simulink library "halout"  (R2021b)
settings: Solver=VariableStepAuto  StartTime=0.0  StopTime=10.0  RelTol=1e-3
undefined symbols (not defined in the file): C_TASK_5MS_S, KHAL_CAN1TxReq_flg, KHAL_CAN2TxReq_flg, KHAL_CAN3TxReq_flg, KHAL_CAN4TxReq_flg, KHAL_CAN5TxReq_flg, KHAL_CAN6TxReq_flg, KHAL_CAN7TxReq_flg, TRUE
libraries: FVT_lib x65, simulink x6
(part 6 of 6)

== system halout/HAL_OUT/CAN4/FD4_CE100_0_0x209/FDCBCMMDCloseSVCmd ==
  FDCBCMMDCloseSVCmd : Inport
  Data Type Conversion : DataTypeConversion  OutDataTypeStr=uint8  RndMeth=Round
  CAN4_FDC_BCM_MDCloseSV_Cmd : Outport
  wires:
  Data Type Conversion/1 -> CAN4_FDC_BCM_MDCloseSV_Cmd/1
  FDCBCMMDCloseSVCmd/1 -> Data Type Conversion/1

== system halout/HAL_OUT/CAN4/FD4_CE100_0_0x209/FDCBCMMDOpenSVCmd ==
  FDCBCMMDOpenSVCmd : Inport
  Data Type Conversion : DataTypeConversion  OutDataTypeStr=uint8  RndMeth=Round
  CAN4_FDC_BCM_MDOpenSV_Cmd : Outport
  wires:
  Data Type Conversion/1 -> CAN4_FDC_BCM_MDOpenSV_Cmd/1
  FDCBCMMDOpenSVCmd/1 -> Data Type Conversion/1

== system halout/HAL_OUT/CAN4/FD4_CE100_0_0x209/FDCBCMMDoorSta ==
  FDCBCMMDoorSta : Inport
  Data Type Conversion : DataTypeConversion  OutDataTypeStr=uint8  RndMeth=Round
  CAN4_FDC_BCM_MDoor_Sta : Outport
  wires:
  Data Type Conversion/1 -> CAN4_FDC_BCM_MDoor_Sta/1
  FDCBCMMDoorSta/1 -> Data Type Conversion/1

== system halout/HAL_OUT/CAN4/FD4_CE100_0_0x209/FDCBCMOutDoorOpenSWSta ==
  FDCBCMOutDoorOpenSWSta : Inport
  Data Type Conversion : DataTypeConversion  OutDataTypeStr=uint8  RndMeth=Round
  CAN4_FDC_BCM_OutDoorOpenSW_Sta : Outport
  wires:
  Data Type Conversion/1 -> CAN4_FDC_BCM_OutDoorOpenSW_Sta/1
  FDCBCMOutDoorOpenSWSta/1 -> Data Type Conversion/1

== system halout/HAL_OUT/CAN4/FD4_CE100_0_0x209/FDCBCMPLampCmd ==
  FDCBCMPLampCmd : Inport
  Data Type Conversion : DataTypeConversion  OutDataTypeStr=uint8  RndMeth=Round
  CAN4_FDC_BCM_PLamp_Cmd : Outport
  wires:
  Data Type Conversion/1 -> CAN4_FDC_BCM_PLamp_Cmd/1
  FDCBCMPLampCmd/1 -> Data Type Conversion/1

== system halout/HAL_OUT/CAN4/FD4_CE100_0_0x209/FDCBCMRBSDRCmd ==
  FDCBCMRBSDRCmd : Inport
  Data Type Conversion : DataTypeConversion  OutDataTypeStr=uint8  RndMeth=Round
  CAN4_FDC_BCM_RBSDR_Cmd : Outport
  wires:
  Data Type Conversion/1 -> CAN4_FDC_BCM_RBSDR_Cmd/1
  FDCBCMRBSDRCmd/1 -> Data Type Conversion/1

== system halout/HAL_OUT/CAN4/FD4_CE100_0_0x209/FDCBCMRBSDYCmd ==
  FDCBCMRBSDYCmd : Inport
  Data Type Conversion : DataTypeConversion  OutDataTypeStr=uint8  RndMeth=Round
  CAN4_FDC_BCM_RBSDY_Cmd : Outport
  wires:
  Data Type Conversion/1 -> CAN4_FDC_BCM_RBSDY_Cmd/1
  FDCBCMRBSDYCmd/1 -> Data Type Conversion/1

== system halout/HAL_OUT/CAN4/FD4_CE100_0_0x209/FDCBCMRDRLCmd ==
  FDCBCMRDRLCmd : Inport
  Data Type Conversion : DataTypeConversion  OutDataTypeStr=uint8  RndMeth=Round
  CAN4_FDC_BCM_RDRL_Cmd : Outport
  wires:
  Data Type Conversion/1 -> CAN4_FDC_BCM_RDRL_Cmd/1
  FDCBCMRDRLCmd/1 -> Data Type Conversion/1

== system halout/HAL_OUT/CAN4/FD4_CE100_0_0x209/FDCBCMRDoorSta ==
  FDCBCMRDoorSta : Inport
  Data Type Conversion : DataTypeConversion  OutDataTypeStr=uint8  RndMeth=Round
  CAN4_FDC_BCM_RDoor_Sta : Outport
  wires:
  Data Type Conversion/1 -> CAN4_FDC_BCM_RDoor_Sta/1
  FDCBCMRDoorSta/1 -> Data Type Conversion/1

== system halout/HAL_OUT/CAN4/FD4_CE100_0_0x209/FDCBCMRFLampCmd ==
  FDCBCMRFLampCmd : Inport
  Data Type Conversion : DataTypeConversion  OutDataTypeStr=uint8  RndMeth=Round
  CAN4_FDC_BCM_RFLamp_Cmd : Outport
  wires:
  Data Type Conversion/1 -> CAN4_FDC_BCM_RFLamp_Cmd/1
  FDCBCMRFLampCmd/1 -> Data Type Conversion/1

== system halout/HAL_OUT/CAN4/FD4_CE100_0_0x209/FDCBCMRGearSta ==
  FDCBCMRGearSta : Inport
  Data Type Conversion : DataTypeConversion  OutDataTypeStr=uint8  RndMeth=Round
  CAN4_FDC_BCM_RGear_Sta : Outport
  wires:
  Data Type Conversion/1 -> CAN4_FDC_BCM_RGear_Sta/1
  FDCBCMRGearSta/1 -> Data Type Conversion/1

== system halout/HAL_OUT/CAN4/FD4_CE100_0_0x209/FDCBCMRTurnLpCmd ==
  FDCBCMRTurnLpCmd : Inport
  Data Type Conversion : DataTypeConversion  OutDataTypeStr=uint8  RndMeth=Round
  CAN4_FDC_BCM_RTurnLp_Cmd : Outport
  wires:
  Data Type Conversion/1 -> CAN4_FDC_BCM_RTurnLp_Cmd/1
  FDCBCMRTurnLpCmd/1 -> Data Type Conversion/1

== system halout/HAL_OUT/CAN4/FD4_CE100_0_0x209/FDCBCMRoomLpAmbCmd ==
  FDCBCMRoomLpAmbCmd : Inport
  Data Type Conversion : DataTypeConversion  OutDataTypeStr=uint8  RndMeth=Round
  CAN4_FDC_BCM_RoomLpAmb_Cmd : Outport
  wires:
  Data Type Conversion/1 -> CAN4_FDC_BCM_RoomLpAmb_Cmd/1
  FDCBCMRoomLpAmbCmd/1 -> Data Type Conversion/1

== system halout/HAL_OUT/CAN4/FD4_CE100_0_0x209/FDCBCMSLTLpCmd ==
  FDCBCMSLTLpCmd : Inport
  Data Type Conversion : DataTypeConversion  OutDataTypeStr=uint8  RndMeth=Round
  CAN4_FDC_BCM_SLTLp_Cmd : Outport
  wires:
  Data Type Conversion/1 -> CAN4_FDC_BCM_SLTLp_Cmd/1
  FDCBCMSLTLpCmd/1 -> Data Type Conversion/1

== system halout/HAL_OUT/CAN4/FD4_CE100_0_0x209/FDCBCMSMKLCmd ==
  FDCBCMSMKLCmd : Inport
  Data Type Conversion : DataTypeConversion  OutDataTypeStr=uint8  RndMeth=Round
  CAN4_FDC_BCM_SMKL_Cmd : Outport
  wires:
  Data Type Conversion/1 -> CAN4_FDC_BCM_SMKL_Cmd/1
  FDCBCMSMKLCmd/1 -> Data Type Conversion/1

== system halout/HAL_OUT/CAN4/FD4_CE100_0_0x209/FDCBCMSMKRCmd ==
  FDCBCMSMKRCmd : Inport
  Data Type Conversion : DataTypeConversion  OutDataTypeStr=uint8  RndMeth=Round
  CAN4_FDC_BCM_SMKR_Cmd : Outport
  wires:
  Data Type Conversion/1 -> CAN4_FDC_BCM_SMKR_Cmd/1
  FDCBCMSMKRCmd/1 -> Data Type Conversion/1

== system halout/HAL_OUT/CAN4/FD4_CE100_0_0x209/FDCBCMSRTLpCmd ==
  FDCBCMSRTLpCmd : Inport
  Data Type Conversion : DataTypeConversion  OutDataTypeStr=uint8  RndMeth=Round
  CAN4_FDC_BCM_SRTLp_Cmd : Outport
  wires:
  Data Type Conversion/1 -> CAN4_FDC_BCM_SRTLp_Cmd/1
  FDCBCMSRTLpCmd/1 -> Data Type Conversion/1

== system halout/HAL_OUT/CAN4/FD4_CE100_0_0x209/FDCBCMSTOPBALLCmd ==
  FDCBCMSTOPBALLCmd : Inport
  Data Type Conversion : DataTypeConversion  OutDataTypeStr=uint8  RndMeth=Round
  CAN4_FDC_BCM_STOPBALL_Cmd : Outport
  wires:
  Data Type Conversion/1 -> CAN4_FDC_BCM_STOPBALL_Cmd/1
  FDCBCMSTOPBALLCmd/1 -> Data Type Conversion/1

== system halout/HAL_OUT/CAN4/FD4_CE100_0_0x209/FDCBCMStopINDCmd ==
  FDCBCMStopINDCmd : Inport
  Data Type Conversion : DataTypeConversion  OutDataTypeStr=uint8  RndMeth=Round
  CAN4_FDC_BCM_Stop_IND_Cmd : Outport
  wires:
  Data Type Conversion/1 -> CAN4_FDC_BCM_Stop_IND_Cmd/1
  FDCBCMStopINDCmd/1 -> Data Type Conversion/1

== system halout/HAL_OUT/CAN4/FD4_CE100_0_0x209/FDCBCMTurnLpPatternSta ==
  FDCBCMTurnLpPatternSta : Inport
  Data Type Conversion : DataTypeConversion  OutDataTypeStr=uint8  RndMeth=Round
  CAN4_FDC_BCM_TurnLpPattern_Sta : Outport
  wires:
  Data Type Conversion/1 -> CAN4_FDC_BCM_TurnLpPattern_Sta/1
  FDCBCMTurnLpPatternSta/1 -> Data Type Conversion/1

== system halout/HAL_OUT/CAN4/FD4_CE100_0_0x209/FDCBCMWasherCmd ==
  FDCBCMWasherCmd : Inport
  Data Type Conversion : DataTypeConversion  OutDataTypeStr=uint8  RndMeth=Round
  CAN4_FDC_BCM_Washer_Cmd : Outport
  wires:
  Data Type Conversion/1 -> CAN4_FDC_BCM_Washer_Cmd/1
  FDCBCMWasherCmd/1 -> Data Type Conversion/1

== system halout/HAL_OUT/CAN4/FD4_CE100_0_0x209/FDCBCMWiperHCmd ==
  FDCBCMWiperHCmd : Inport
  Data Type Conversion : DataTypeConversion  OutDataTypeStr=uint8  RndMeth=Round
  CAN4_FDC_BCM_WiperH_Cmd : Outport
  wires:
  Data Type Conversion/1 -> CAN4_FDC_BCM_WiperH_Cmd/1
  FDCBCMWiperHCmd/1 -> Data Type Conversion/1

== system halout/HAL_OUT/CAN4/FD4_CE100_0_0x209/FDCBCMWiperLCmd ==
  FDCBCMWiperLCmd : Inport
  Data Type Conversion : DataTypeConversion  OutDataTypeStr=uint8  RndMeth=Round
  CAN4_FDC_BCM_WiperL_Cmd : Outport
  wires:
  Data Type Conversion/1 -> CAN4_FDC_BCM_WiperL_Cmd/1
  FDCBCMWiperLCmd/1 -> Data Type Conversion/1

== system halout/HAL_OUT/CAN4/FD4_CE100_0_0x209/VCUKeyStatus ==
  VCUKeyStatus : Inport
  Data Type Conversion : DataTypeConversion  OutDataTypeStr=uint8  RndMeth=Round
  CAN4_VCUKeyStatus : Outport
  wires:
  Data Type Conversion/1 -> CAN4_VCUKeyStatus/1
  VCUKeyStatus/1 -> Data Type Conversion/1

== system halout/HAL_OUT/CAN4/FD4_CE100_1_0x210/FDCBCMFRoomLpCmd ==
  FDCBCMFRoomLpCmd : Inport
  Data Type Conversion : DataTypeConversion  OutDataTypeStr=uint8  RndMeth=Round
  CAN4_FDC_BCM_FRoomLp_Cmd : Outport
  wires:
  Data Type Conversion/1 -> CAN4_FDC_BCM_FRoomLp_Cmd/1
  FDCBCMFRoomLpCmd/1 -> Data Type Conversion/1

== system halout/HAL_OUT/CAN4/FD4_CE100_1_0x210/FDCBCMMRoomLpCmd ==
  FDCBCMMRoomLpCmd : Inport
  Data Type Conversion : DataTypeConversion  OutDataTypeStr=uint8  RndMeth=Round
  CAN4_FDC_BCM_MRoomLp_Cmd : Outport
  wires:
  Data Type Conversion/1 -> CAN4_FDC_BCM_MRoomLp_Cmd/1
  FDCBCMMRoomLpCmd/1 -> Data Type Conversion/1

== system halout/HAL_OUT/CAN4/FD4_CE100_1_0x210/FDCBCMRRoomLpCmd ==
  FDCBCMRRoomLpCmd : Inport
  Data Type Conversion : DataTypeConversion  OutDataTypeStr=uint8  RndMeth=Round
  CAN4_FDC_BCM_RRoomLp_Cmd : Outport
  wires:
  Data Type Conversion/1 -> CAN4_FDC_BCM_RRoomLp_Cmd/1
  FDCBCMRRoomLpCmd/1 -> Data Type Conversion/1

== system halout/HAL_OUT/CAN4/FD4_CE100_1_0x210/FDCTHCMCoolFanReqCmd ==
  FDCTHCMCoolFanReqCmd : Inport
  Data Type Conversion : DataTypeConversion  OutDataTypeStr=uint8  RndMeth=Round
  convert_out : FVT_lib/hal/convert_out  gain=0.5  offset=0
  CAN4_FDC_THCM_CoolFanReq_Cmd : Outport
  wires:
  Data Type Conversion/1 -> CAN4_FDC_THCM_CoolFanReq_Cmd/1
  convert_out/1 -> Data Type Conversion/1
  FDCTHCMCoolFanReqCmd/1 -> convert_out/1

== system halout/HAL_OUT/CAN5/FD5_C100_0_0x18F348D0/AlcLockSta ==
  AlcLockSta : Inport
  Data Type Conversion : DataTypeConversion  OutDataTypeStr=uint8  RndMeth=Round
  CAN5_AlcLockSta : Outport
  wires:
  Data Type Conversion/1 -> CAN5_AlcLockSta/1
  AlcLockSta/1 -> Data Type Conversion/1

== system halout/HAL_OUT/CAN5/FD5_C100_0_0x18F348D0/B2VAPlusSta ==
  B2VAPlusSta : Inport
  Data Type Conversion : DataTypeConversion  OutDataTypeStr=uint8  RndMeth=Round
  CAN5_B2VAPlusSta : Outport
  wires:
  Data Type Conversion/1 -> CAN5_B2VAPlusSta/1
  B2VAPlusSta/1 -> Data Type Conversion/1

== system halout/HAL_OUT/CAN5/FD5_C100_0_0x18F348D0/VCUHVILSta ==
  VCUHVILSta : Inport
  Data Type Conversion : DataTypeConversion  OutDataTypeStr=uint8  RndMeth=Round
  CAN5_VCUHVILSta : Outport
  wires:
  Data Type Conversion/1 -> CAN5_VCUHVILSta/1
  VCUHVILSta/1 -> Data Type Conversion/1

== system halout/HAL_OUT/CAN5/FD5_C200_0_0x20D/SysPowerMode ==
  SysPowerMode : Inport
  Data Type Conversion : DataTypeConversion  OutDataTypeStr=uint8  RndMeth=Round
  CAN5_SysPowerMode : Outport
  wires:
  Data Type Conversion/1 -> CAN5_SysPowerMode/1
  SysPowerMode/1 -> Data Type Conversion/1

== system halout/HAL_OUT/CAN6/FD6_C200_0_0x20C/SysPowerMode ==
  SysPowerMode : Inport
  Data Type Conversion : DataTypeConversion  OutDataTypeStr=uint8  RndMeth=Round
  CAN6_SysPowerMode : Outport
  wires:
  Data Type Conversion/1 -> CAN6_SysPowerMode/1
  SysPowerMode/1 -> Data Type Conversion/1

== system halout/HAL_OUT/CAN7/FD7_C100_0_0x19F005D0/VCUKeyStatus ==
  VCUKeyStatus : Inport
  Data Type Conversion : DataTypeConversion  OutDataTypeStr=uint8  RndMeth=Round
  CAN7_VCUKeyStatus : Outport
  wires:
  Data Type Conversion/1 -> CAN7_VCUKeyStatus/1
  VCUKeyStatus/1 -> Data Type Conversion/1

== system halout/HAL_OUT/CAN7/FD7_C10_0_0xC61D0D1/EMotorSpd ==
  EMotorSpd : Inport
  Data Type Conversion : DataTypeConversion  OutDataTypeStr=uint16  RndMeth=Round
  CAN7_EMotorSpd : Outport
  wires:
  Data Type Conversion/1 -> CAN7_EMotorSpd/1
  EMotorSpd/1 -> Data Type Conversion/1

== system halout/HAL_OUT/CAN7/FD7_C200_0_0x18F003EF/SysPowerMode ==
  SysPowerMode : Inport
  Data Type Conversion : DataTypeConversion  OutDataTypeStr=uint8  RndMeth=Round
  CAN7_SysPowerMode : Outport
  wires:
  Data Type Conversion/1 -> CAN7_SysPowerMode/1
  SysPowerMode/1 -> Data Type Conversion/1

== system halout/HAL_OUT/CAN7/FD7_C50_0_0xCF00300/AccPedalPos1 ==
  AccPedalPos1 : Inport
  Data Type Conversion : DataTypeConversion  OutDataTypeStr=uint8  RndMeth=Round
  convert_out : FVT_lib/hal/convert_out  gain=0.4  offset=0
  CAN7_AccPedalPos1 : Outport
  wires:
  Data Type Conversion/1 -> CAN7_AccPedalPos1/1
  convert_out/1 -> Data Type Conversion/1
  AccPedalPos1/1 -> convert_out/1

== system halout/HAL_OUT/CAN7/FD7_CE100_0_0x18FA05B9/FDCBCMDVRSignalLCmd ==
  FDCBCMDVRSignalLCmd : Inport
  Data Type Conversion : DataTypeConversion  OutDataTypeStr=uint8  RndMeth=Round
  CAN7_FDC_BCM_DVRSignalL_Cmd : Outport
  wires:
  Data Type Conversion/1 -> CAN7_FDC_BCM_DVRSignalL_Cmd/1
  FDCBCMDVRSignalLCmd/1 -> Data Type Conversion/1

== system halout/HAL_OUT/CAN7/FD7_CE100_0_0x18FA05B9/FDCBCMDVRSignalRCmd ==
  FDCBCMDVRSignalRCmd : Inport
  Data Type Conversion : DataTypeConversion  OutDataTypeStr=uint8  RndMeth=Round
  CAN7_FDC_BCM_DVRSignalR_Cmd : Outport
  wires:
  Data Type Conversion/1 -> CAN7_FDC_BCM_DVRSignalR_Cmd/1
  FDCBCMDVRSignalRCmd/1 -> Data Type Conversion/1

== system halout/HAL_OUT/CAN7/FD7_CE100_0_0x18FA05B9/FDCBCMFDoorSta ==
  FDCBCMFDoorSta : Inport
  Data Type Conversion : DataTypeConversion  OutDataTypeStr=uint8  RndMeth=Round
  CAN7_FDC_BCM_FDoor_Sta : Outport
  wires:
  Data Type Conversion/1 -> CAN7_FDC_BCM_FDoor_Sta/1
  FDCBCMFDoorSta/1 -> Data Type Conversion/1

== system halout/HAL_OUT/CAN7/FD7_CE100_0_0x18FA05B9/FDCBCMHBeamCmd ==
  FDCBCMHBeamCmd : Inport
  Data Type Conversion : DataTypeConversion  OutDataTypeStr=uint8  RndMeth=Round
  CAN7_FDC_BCM_HBeam_Cmd : Outport
  wires:
  Data Type Conversion/1 -> CAN7_FDC_BCM_HBeam_Cmd/1
  FDCBCMHBeamCmd/1 -> Data Type Conversion/1

== system halout/HAL_OUT/CAN7/FD7_CE100_0_0x18FA05B9/FDCBCMLBeamCmd ==
  FDCBCMLBeamCmd : Inport
  Data Type Conversion : DataTypeConversion  OutDataTypeStr=uint8  RndMeth=Round
  CAN7_FDC_BCM_LBeam_Cmd : Outport
  wires:
  Data Type Conversion/1 -> CAN7_FDC_BCM_LBeam_Cmd/1
  FDCBCMLBeamCmd/1 -> Data Type Conversion/1

== system halout/HAL_OUT/CAN7/FD7_CE100_0_0x18FA05B9/FDCBCMMDoorSta ==
  FDCBCMMDoorSta : Inport
  Data Type Conversion : DataTypeConversion  OutDataTypeStr=uint8  RndMeth=Round
  CAN7_FDC_BCM_MDoor_Sta : Outport
  wires:
  Data Type Conversion/1 -> CAN7_FDC_BCM_MDoor_Sta/1
  FDCBCMMDoorSta/1 -> Data Type Conversion/1

== system halout/HAL_OUT/CAN7/FD7_CE100_0_0x18FA05B9/FDCBCMPLampCmd ==
  FDCBCMPLampCmd : Inport
  Data Type Conversion : DataTypeConversion  OutDataTypeStr=uint8  RndMeth=Round
  CAN7_FDC_BCM_PLamp_Cmd : Outport
  wires:
  Data Type Conversion/1 -> CAN7_FDC_BCM_PLamp_Cmd/1
  FDCBCMPLampCmd/1 -> Data Type Conversion/1

== stateflow chart halout/HAL_OUT/CAN3/FD3_VCU2_Tx/Chart ==
  state TrigCounter
    en:
    counter = 0;
    counter++;
    (default) -> (junction 5)
    TrigCounter -> (junction 5) : {
        | counter++;
        | }
    (junction 5) -> (junction 6) [order 1] : [TxReq && (counter %% CycleCnt) == 0]
    (junction 5) -> (junction 7) [order 2]
    (junction 6) -> (junction 8) : {
        | TxTrigger;
        | counter = 0;
        | }
    (junction 8) -> (junction 7)
    (junction 7) -> (junction 34)
    (junction 34) -> (junction 33) [order 1] : [ !TxReq]
    (junction 34) -> (junction 35) [order 2]
    (junction 33) -> (junction 36) : {
        | counter = 0;
        | }
    (junction 36) -> (junction 35)
    (junction 35) -> (junction 44)
  data: TxReq input; CycleCnt input; counter local uint16
  events: TxTrigger output FUNCTION_CALL_EVENT

== stateflow chart halout/HAL_OUT/CAN3/FD3_C10_1_0xCFF05EF/CRC_TX/Checksum_J1939_SPN4207 ==
  (default) -> (junction 2) : {
      | ChecksumLocal = (Byte1+Byte2+Byte3+Byte4+Byte5+Byte6+Byte7)...
      | +(MsgCntLocal & 0x0F)...
      | + (MsgIDLowByte + MsgIDMidLowByte + MsgIDMidHighByte + MsgIDHighByte);
      | }
  (junction 2) -> (junction 5)
  (junction 5) -> (junction 7) : {
      | MsgChecksumLocal = (((ChecksumLocal>>6) & 0x03)...
      | + (ChecksumLocal>>3)...
      | + ChecksumLocal)...
      | & 0x07;
      | }
  data: Byte1 input; Byte2 input; Byte3 input; Byte4 input; Byte5 input; Byte6 input; Byte7 input; MsgCntLocal input; MsgIDLowByte input; MsgIDMidLowByte input; MsgIDMidHighByte input; MsgIDHighByte input; MsgChecksumLocal output uint8; ChecksumLocal local single

== stateflow chart halout/HAL_OUT/CAN3/FD3_C10_1_0xCFF05EF/CRC_TX/Rolling_Counter ==
  state RollingCounter
    en:
    MsgCntLocal = 0;
    RollingCounter -> (junction 2) : {MsgCntLocal ++;}
    (junction 2) -> (junction 4) [order 1] : [MsgCntLocal > 0x07]
    (junction 2) -> (junction 6) [order 2]
    (junction 4) -> (junction 8) : {MsgCntLocal = 0;}
  data: MsgCntLocal output uint8

== stateflow chart halout/HAL_OUT/CAN_Scheduler ==
  state CAN_scheduler
    (default) -> (junction 55)
    CAN_scheduler -> (junction 55)
    (junction 55) -> (junction 53) [order 1] : [KHAL_CAN1TxReq_flg && VOUTP_ALLCANTxReq_flg]
    (junction 55) -> (junction 214) [order 2]
    (junction 53) -> (junction 212) : {
        | trig_can1;
        | }
    (junction 212) -> (junction 214)
    (junction 214) -> (junction 250)
    (junction 250) -> (junction 251) [order 1] : [KHAL_CAN2TxReq_flg && VOUTP_ALLCANTxReq_flg]
    (junction 250) -> (junction 253) [order 2]
    (junction 251) -> (junction 247) : {
        | trig_can2;
        | }
    (junction 247) -> (junction 253)
    (junction 253) -> (junction 258)
    (junction 258) -> (junction 259) [order 1] : [KHAL_CAN3TxReq_flg && VOUTP_ALLCANTxReq_flg]
    (junction 258) -> (junction 261) [order 2]
    (junction 259) -> (junction 255) : {
        | trig_can3;
        | }
    (junction 255) -> (junction 261)
    (junction 261) -> (junction 266)
    (junction 266) -> (junction 267) [order 1] : [KHAL_CAN4TxReq_flg && VOUTP_ALLCANTxReq_flg]
    (junction 266) -> (junction 269) [order 2]
    (junction 267) -> (junction 263) : {
        | trig_can4;
        | }
    (junction 263) -> (junction 269)
    (junction 269) -> (junction 274)
    (junction 274) -> (junction 275) [order 1] : [KHAL_CAN5TxReq_flg && VOUTP_ALLCANTxReq_flg]
    (junction 274) -> (junction 277) [order 2]
    (junction 275) -> (junction 271) : {
        | trig_can5;
        | }
    (junction 271) -> (junction 277)
    (junction 277) -> (junction 323)
    (junction 323) -> (junction 322) [order 1] : [KHAL_CAN6TxReq_flg && VOUTP_ALLCANTxReq_flg]
    (junction 323) -> (junction 324) [order 2]
    (junction 322) -> (junction 321) : {
        | trig_can6;
        | }
    (junction 321) -> (junction 324)
    (junction 324) -> (junction 333)
    (junction 333) -> (junction 339) [order 1] : [KHAL_CAN7TxReq_flg && VOUTP_ALLCANTxReq_flg]
    (junction 333) -> (junction 334) [order 2]
    (junction 339) -> (junction 335) : {
        | trig_can7;
        | }
    (junction 335) -> (junction 334)
  data: KHAL_CAN1TxReq_flg input; KHAL_CAN2TxReq_flg input; KHAL_CAN3TxReq_flg input; KHAL_CAN4TxReq_flg input; KHAL_CAN5TxReq_flg input; KHAL_CAN6TxReq_flg input; KHAL_CAN7TxReq_flg input; VOUTP_ALLCANTxReq_flg input
  events: trig_can1 output FUNCTION_CALL_EVENT; trig_can2 output FUNCTION_CALL_EVENT; trig_can3 output FUNCTION_CALL_EVENT; trig_can4 output FUNCTION_CALL_EVENT; trig_can5 output FUNCTION_CALL_EVENT; trig_can6 output FUNCTION_CALL_EVENT; trig_can7 output FUNCTION_CALL_EVENT
